simulink library "pil_demo_lib"  (Simulink 7.6)
settings: Solver=ode45  SolverMode=SingleTasking  StartTime=0.0  StopTime=10.0  RelTol=1e-3
settings Model: Creator=The MathWorks Inc.  ExtModeAutoUpdateStatusClock=off

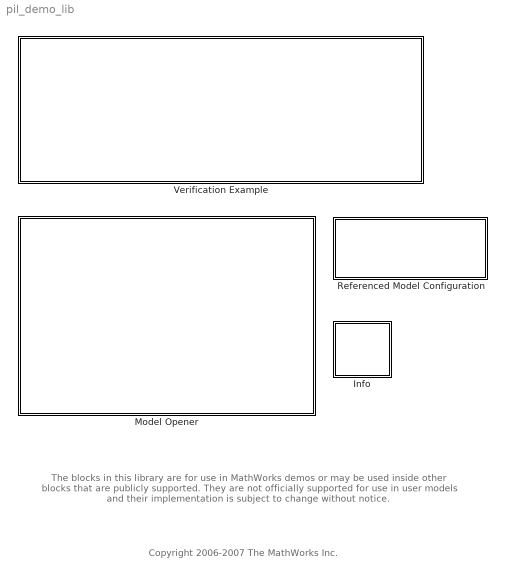
== system pil_demo_lib ==
  note: Copyright 2006-2007 The MathWorks Inc.
  note: The blocks in this library are for use in MathWorks demos or may
      | be used inside other blocks that are publicly supported.
      | They are not officially supported for use in user models
      | and their implementation is subject to change without notice.
  Info : Subsystem
      settings: OpenFcn=showdemo(bdroot(gcb));
      mask Type: Info
      mask Display: image(imread('targets_demo_info.bmp','bmp'),'center')
  Model Opener : Subsystem  mask{modelName=model_based_deployment, modelDescription=Target Processor 2}
      mask prompts: modelName "Model name"; modelDescription "Model description"
      settings: OpenFcn=|
      | modelName = get_param(gcb,'modelName');
      | open_system(modelName);
      mask Display: disp(sprintf('%s\n(double-click to open)\n\n\n\n\n\n\n', modelDescription));
  Referenced Model Configuration : Subsystem  mask(Configure Referenced Model){csDescription=Simulation, thisConfigSet=SIL, models={'alg2'}, configSets={'SIL'}}
      mask prompts: csDescription "Configuration Description"; thisConfigSet "Configuration Set in this Model"; models "Referenced Models"; configSets "Corresponding Configuration Sets"
      settings: OpenFcn=|
      | block = gcb;
      | thisModel = bdroot(gcs);
      | % indicate an action is happening
      | set_param(block, 'BackgroundColor', 'red');
      | try
      | thisConfigSet = get_param(block, 'thisConfigSet');
      | 
      | models = get_param(block, 'models');
      | % Need to evaluate, but avoid slResolve
      | models = eval(models);
      | configSets = get_param(block, 'configSets');
      | % Need to evaluate, but avoid slResolve
      | configSets = eval(configSets);
      | 
      | pil_demo_configure_referenced_models(thisModel, thisConfigSet, models, configSets);
      | catch e                                                                 % restore background
      |    set_param(block, 'BackgroundColor', 'lightBlue');
      |    rethrow(e);
      | end
      | pause(0.5);                                                    % restore background
      | set_param(block, 'BackgroundColor', 'lightBlue');
      mask Display: disp(sprintf('Double-click to\nConfigure Model\nfor %s', csDescription));
  Verification Example : Subsystem  mask{targetBlock=untitled/PIL Block, simulationBlock=algmodel/Alg Block}
      mask prompts: targetBlock "PIL block"; simulationBlock "Simulation block"
      settings: OpenFcn=pil_demo_verify_callback(gcb);
      mask Display: disp(sprintf('An Example Verification Process using "target_block_verify"\n\n\nDouble-click to verify:\n\nSimulation block: %s\nTarget block: %s', simulationBlock, targetBlock));

== system pil_demo_lib/Info ==

== system pil_demo_lib/Model Opener ==

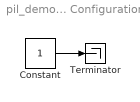
== system pil_demo_lib/Referenced Model Configuration ==
  Constant : Constant  OutDataTypeStr=uint8
  Terminator : Terminator
  wires:
  Constant/1 -> Terminator/1

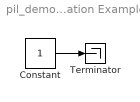
== system pil_demo_lib/Verification Example ==
  Constant : Constant  OutDataTypeStr=uint8
  Terminator : Terminator
  wires:
  Constant/1 -> Terminator/1
